simulink model "power_filter"  (Simulink 6.0)
settings: Solver=ode45  SolverMode=SingleTasking  StartTime=0.0  StopTime=0.1  RelTol=1e-3  AbsTol=1e-6
libraries: powerlib x8
settings Model: Creator=patrice  LastModifiedBy=batserve  ExtModeTrigMode=oneshot  ExtModeArmWhenConnect=off  ExtModeAutoUpdateStatusClock=off
settings DataIOCC: LimitDataPoints=off  SignalLoggingName=sigsOut
settings OptimizationCC: BlockReduction=off  BooleanDataType=off
settings DebuggingCC: CheckExecutionContextPreStartOutputMsg=on  CheckExecutionContextRuntimeOutputMsg=on  SolverPrmCheckMsg=none
settings HardwareCC: TargetUnknown=on
settings RTWCC: TemplateMakefile=grt_unix.tmf

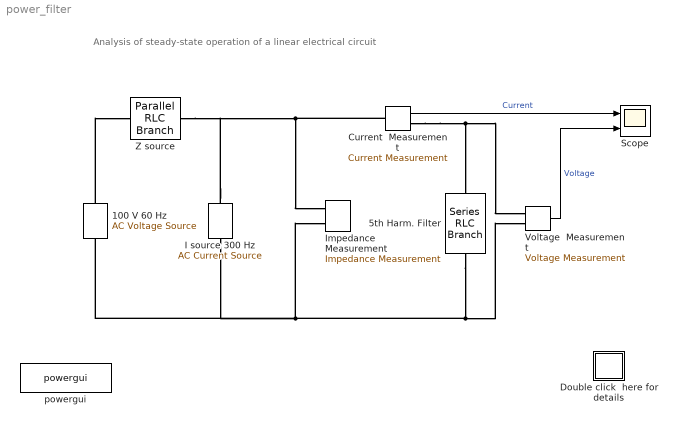
== system power_filter ==
  note: Analysis of steady-state operation of a linear electrical circuit
  100 V 60 Hz : powerlib/Electrical Sources/AC Voltage Source  Description=source block  Orientation=up  Amplitude=100  Phase=0  Frequency=60  SampleTime=0  Measurements=None
      settings: AttributesFormatString=\n
  5th Harm. Filter : powerlib/Elements/Series RLC Branch  Orientation=down  PhysicalDomain=powersysdomain  SubClassName=unknown  LeftPortType=p1  RightPortType=p1  LConnTagsString=__new0  RConnTagsString=__new0  Resistance=1.27  Inductance=107.42e-03  Capacitance=2.62e-06  Measurements=None
  Current  Measurement : powerlib/Measurements/Current Measurement  Tag=PoWeRsYsTeMmEaSuReMeNt  PhasorSimulation=off  OutputType=Magnitude  PSBequivalent=0
  Double click  here for details : Subsystem
      mask Display: disp('?')
  I source 300 Hz : powerlib/Electrical Sources/AC Current Source  Orientation=up  Amplitude=10  Phase=-30  Frequency=300  SampleTime=0  Measurements=None
      settings: AttributesFormatString=\n
  Impedance  Measurement : powerlib/Measurements/Impedance Measurement  PhysicalDomain=powersysdomain  SubClassName=unknown  LeftPortType=p1  RightPortType=p1  LConnTagsString=+|-  Factor=1
      settings: AttributesFormatString=\n
  Scope : Scope  NumInputPorts=2
      settings: TimeRange=0.1  YMin=-10~-200  YMax=10~200  DataFormat=Array
  Voltage  Measurement : powerlib/Measurements/Voltage Measurement  Tag=PoWeRsYsTeMmEaSuReMeNt  PhasorSimulation=off  OutputType=Magnitude  PSBequivalent=0
  Z source : powerlib/Elements/Parallel RLC Branch  PhysicalDomain=powersysdomain  SubClassName=unknown  LeftPortType=p1  RightPortType=p1  LConnTagsString=a  RConnTagsString=__new0  Resistance=37.7  Inductance=10e-03  Capacitance=0  Measurements=None
  powergui : powerlib/powergui  Priority=2  Frange=0:2:1000  Ylog=off  Xlog=off  save=off  variable=ZData  ZoomFFT=on  StartTime=0.0  cycles=1  DisplayStyle=off  fundamental=60  FreqAxis=off  MaxFrequency=1000  frequencyindice=1  frequencyindicesteady=1  RmsSteady=1  display=off  Ts=0  methode=off  frequency=60  echomessages=on
  wires:
  Current  Measurement/1 -> Scope/1  "Current"
  Voltage  Measurement/1 -> Scope/2  "Voltage"
  connections:
  100 V 60 Hz/RConn1 -- Z source/LConn1
  Current  Measurement/LConn1 -- I source 300 Hz/RConn1 -- Z source/RConn1 -- Impedance  Measurement/LConn1
  5th Harm. Filter/RConn1 -- Impedance  Measurement/LConn2 -- I source 300 Hz/LConn1 -- 100 V 60 Hz/LConn1 -- Voltage  Measurement/LConn2
  Current  Measurement/RConn1 -- 5th Harm. Filter/LConn1 -- Voltage  Measurement/LConn1

== system power_filter/Double click  here for details ==
  note: 3
  note: 1
  note: Circuit Description
  note: Demonstration
  note: 2
  note: This demonstration illustrates use of the Powergui
      | and Impedance Measurement blocks to analyze the
      | steady-state operation of a linear electrical circuit
  note: Use the Powergui block to find the steady-sate  60Hz  and 300 Hz  components of  voltage and
      | current phasors.  The values of the 3 states (phasors and initial values)  can be also obtained
      | from the powergui block.
      |
      | Open the scope and start the simulation from the Simulation/Start menu.
      | Notice that the simulation starts in steady-state.
      |
      | Using the Powergui block,  select Impedance vs Frequency Measurement. A new window opens.
      |
      | The measurement will be performed for the specified frequency range vector [0: 2:1000]  (0 to 1000 Hz
      | by steps of 2 Hz). Click on the Display button. The impedance is dispayed in a graphic window.
      | Notice the series resonance at 300 Hz corresponding to the tuned frequency of the filter.
  note: A 5th harmonic filter is connected at a bus bar fed by a  60 Hz, 100 V inductive source.
      | A 5th harmonic (300 Hz, 1 A) current is injected at the bus bar.
      |
      | This linear system consists of 3 states (2 inductor currents and 1 capacitor voltage),
      |  2 inputs (Vs, Is) and 2 outputs (Current and Voltage Measurement).
      |
      | An Impedance Measurement  block is used to compute the impedance versus frequency of the circuit.
  note: G. Sybille (Hydro-Quebec)
